simulink model "flowchart2"  (R2017b)
settings: Solver=FixedStepDiscrete  StartTime=0.0  StopTime=10.0  FixedStep=1  RelTol=1e-3
model workspace (MAT data in the model file):
  ContractValidatorBlocksMap : containers.Map (value not decoded)
  already_pp = 1
settings Model: Creator=Mudathir  LastModifiedBy=hbourbou
settings OptimizationCC: LifeSpan=inf
settings DebuggingCC: AlgebraicLoopMsg=error  SFExecutionAtInitializationDiag=none
settings HardwareCC: ProdBitPerSizeT=32  ProdBitPerPtrDiffT=32  ProdWordSize=32  ProdHWDeviceType=Specified
settings CodeAppCC: StateflowObjectComments=on

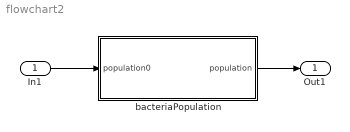
== system flowchart2 ==
  In1 : Inport
  bacteriaPopulation : Stateflow chart  TreatAsAtomicUnit=on
  Out1 : Outport
  wires:
  bacteriaPopulation/1(population) -> Out1/1
  In1/1 -> bacteriaPopulation/1(population0)

== stateflow chart flowchart2/bacteriaPopulation ==
  state start
    entry:
    prePopulation = population0;
    population = population0;
  state state
    (default) -> (junction 128)
    (junction 128) -> (junction 122) [order 1] : [ population < 32.0 ]{prePopulation = population; population = population*2;}
    (junction 128) -> (junction 130) [order 2]
    (junction 130) -> (junction 122) [order 1] : [ population > 32.0 ]{prePopulation = population; ...
        | population = population/2;}
    (junction 122) -> (junction 126) : {disp('efefe')}
    (junction 125) -> (junction 122)
    (junction 130) -> (junction 125) [order 2]
  (default) -> start
  state -> (junction 13)
  start -> (junction 13)
  (junction 13) -> state
  data: population output; population0 input; prePopulation local
  events: dummyEvent local FUNCTION_CALL_EVENT
